simulink model "model_p5"  (R2020b)
settings: Solver=VariableStepAuto  StartTime=0.0  StopTime=10.0  RelTol=1e-3
model workspace (MAT data in the model file):
  C = Simulink.Parameter
  C.Value = 1e-05
  C.DataType = 'auto'
  C.Dimensions = [1 1]
  R = Simulink.Parameter
  R.Value = 10
  R.DataType = 'auto'
  R.Dimensions = [1 1]
settings Model: Creator=ADMIN  LastModifiedBy=ADMIN

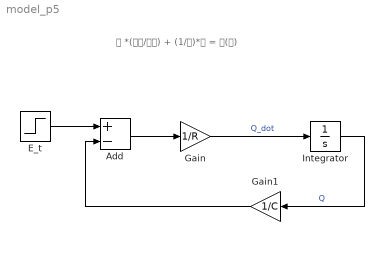
== system model_p5 ==
  note: 𝑅 *(𝑑𝑄/𝑑𝑡) + (1/𝐶)*𝑄 = 𝐸(𝑡)
  Add : Sum  Inputs=+-
  E_t : Step  SampleTime=0
  Gain : Gain  Gain=1/R
  Gain1 : Gain  Gain=1/C
  Integrator : Integrator  InitialCondition=0.00002
  wires:
  Integrator/1 -> Gain1/1  "Q"
  Gain/1 -> Integrator/1  "Q_dot"
  E_t/1 -> Add/1
  Gain1/1 -> Add/2
  Add/1 -> Gain/1
